simulink model "simpletrans"  (R2017a)
settings: Solver=VariableStepAuto  StartTime=0.0  StopTime=100E-6  RelTol=1e-3
libraries: simulink x1, hdlsllib x1
settings Model: Creator=beckmanf  LastModifiedBy=beckmanf
settings OptimizationCC: BlockReduction=off  ConditionallyExecuteInputs=off  DefaultParameterBehavior=Inlined
settings DebuggingCC: AlgebraicLoopMsg=error
settings HardwareCC: ProdBitPerPointer=32  ProdBitPerSizeT=32  ProdBitPerPtrDiffT=32  ProdLargestAtomicFloat=None  ProdIntDivRoundTo=Undefined  ProdEndianess=Unspecified  ProdWordSize=32  ProdHWDeviceType=ASIC/FPGA->ASIC/FPGA  ProdEqTarget=off

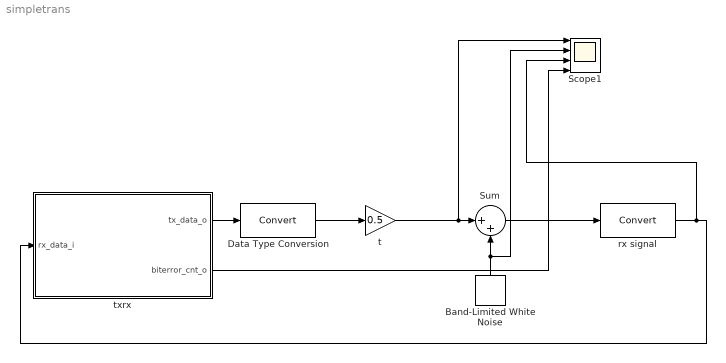
== system simpletrans ==
  Band-Limited White Noise : simulink/Sources/Band-Limited White Noise  Cov=[0.0000000005]  Ts=20E-9  seed=[23341]
  Data Type Conversion : DataTypeConversion
  Scope1 : Scope  NumInputPorts=4
  Sum : Sum  Inputs=|++
  rx signal : DataTypeConversion  SaturateOnIntegerOverflow=on
  t : Gain  Gain=0.5
  txrx : Subsystem
  wires:
  txrx/2(biterror_cnt_o) -> Scope1/4
  txrx/1(tx_data_o) -> Data Type Conversion/1
  Band-Limited White Noise/1 -> Scope1/2, Sum/2
  t/1 -> Scope1/1, Sum/1
  Sum/1 -> rx signal/1
  rx signal/1 -> Scope1/3, txrx/1(rx_data_i)
  Data Type Conversion/1 -> t/1

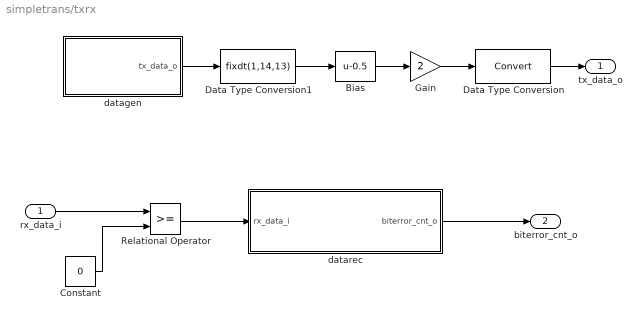
== system simpletrans/txrx ==
  rx_data_i : Inport  OutDataTypeStr=fixdt(1,14,13)
  Bias : Bias  Bias=-0.5
  Constant : Constant  Value=0  OutDataTypeStr=Inherit: Inherit via back propagation
  Data Type Conversion : DataTypeConversion
  Data Type Conversion1 : DataTypeConversion  OutDataTypeStr=fixdt(1,14,13)  SaturateOnIntegerOverflow=on
  Gain : Gain  Gain=2
  Relational Operator : RelationalOperator  OutDataTypeStr=boolean  RndMeth=Nearest
  datagen : Subsystem
  datarec : Subsystem
  tx_data_o : Outport  OutDataTypeStr=fixdt(1,14,13)
  biterror_cnt_o : Outport  Port=2
  wires:
  datagen/1(tx_data_o) -> Data Type Conversion1/1
  datarec/1(biterror_cnt_o) -> biterror_cnt_o/1
  Relational Operator/1 -> datarec/1(rx_data_i)
  Data Type Conversion1/1 -> Bias/1
  Constant/1 -> Relational Operator/2
  rx_data_i/1 -> Relational Operator/1
  Bias/1 -> Gain/1
  Gain/1 -> Data Type Conversion/1
  Data Type Conversion/1 -> tx_data_o/1

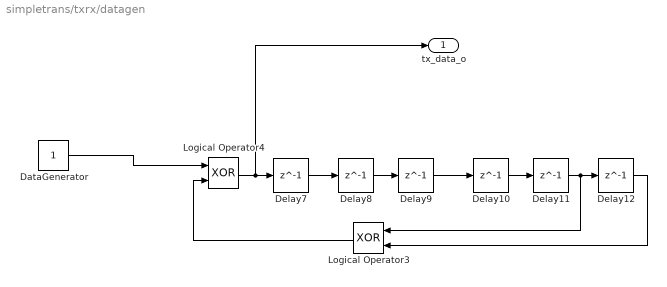
== system simpletrans/txrx/datagen ==
  DataGenerator : Constant  OutDataTypeStr=boolean  SampleTime=20E-9
  Delay{7..11} (5 alike) : Delay  DelayLength=1  InitialCondition=0
  Delay12 : Delay  DelayLength=1  InitialCondition=1
  Logical Operator3 : Logic  Operator=XOR  AllPortsSameDT=off  OutDataTypeStr=boolean
  Logical Operator4 : Logic  Operator=XOR  AllPortsSameDT=off  OutDataTypeStr=boolean
  tx_data_o : Outport
  wires:
  DataGenerator/1 -> Logical Operator4/1
  Logical Operator3/1 -> Logical Operator4/2
  Delay7/1 -> Delay8/1
  Delay9/1 -> Delay10/1
  Delay10/1 -> Delay11/1
  Delay12/1 -> Logical Operator3/2
  Delay11/1 -> Logical Operator3/1, Delay12/1
  Delay8/1 -> Delay9/1
  Logical Operator4/1 -> tx_data_o/1, Delay7/1

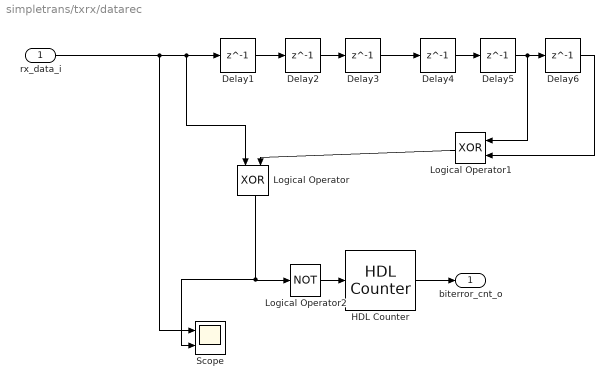
== system simpletrans/txrx/datarec ==
  rx_data_i : Inport  OutDataTypeStr=boolean  PortDimensions=1
  Delay1 : Delay  DelayLength=1  InitialCondition=1
  Delay2 : Delay  DelayLength=1  InitialCondition=1
  Delay{3..6} (4 alike) : Delay  DelayLength=1  InitialCondition=0
  HDL Counter : hdlsllib/HDL Operations/HDL Counter  CountType=Free running  CountInit=0  CountStep=1  CountMax=25  CountFromType=Initial value  CountFrom=0  CountResetPort=off  CountLoadPort=off  CountEnbPort=on  CountDirPort=off  CountDataType=Unsigned  CountWordLen=8  CountFracLen=0  CountSampTime=1
      settings: SourceProductName=HDL Coder  SourceProductBaseCode=HD
  Logical Operator : Logic  Operator=XOR  AllPortsSameDT=off  OutDataTypeStr=boolean
  Logical Operator1 : Logic  Operator=XOR  AllPortsSameDT=off  OutDataTypeStr=boolean
  Logical Operator2 : Logic  Operator=NOT  Inputs=1  AllPortsSameDT=off  OutDataTypeStr=boolean
  Scope : Scope  NumInputPorts=2
  biterror_cnt_o : Outport
  wires:
  rx_data_i/1 -> Scope/1, Logical Operator/1, Delay1/1
  Delay2/1 -> Delay3/1
  Logical Operator1/1 -> Logical Operator/2
  HDL Counter/1 -> biterror_cnt_o/1
  Delay3/1 -> Delay4/1
  Delay6/1 -> Logical Operator1/2
  Delay5/1 -> Logical Operator1/1, Delay6/1
  Logical Operator/1 -> Scope/2, Logical Operator2/1
  Delay1/1 -> Delay2/1
  Delay4/1 -> Delay5/1
  Logical Operator2/1 -> HDL Counter/1
